simulink model "VCU_tb"  (R2023b)
settings: Solver=ode8  StartTime=0.0  StopTime=inf  FixedStep=0.0001  RelTol=1e-3
undefined symbols (not defined in the file or in its folder): canChannel
libraries: fl_lib x3, nesl_utility x3, ee_lib x2, canmsglib x1, canlib x1
settings Model: Creator=rebek  LastModifiedBy=heyka

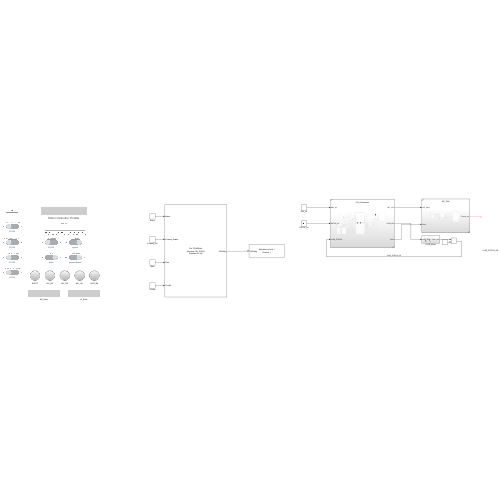
[thumbnail: Simulink's stored preview of the top-level diagram]
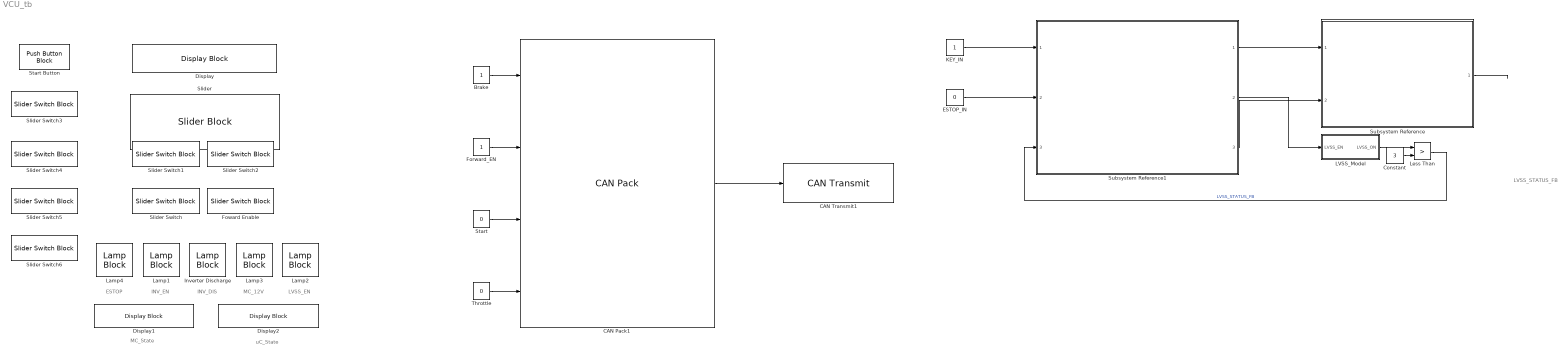
== system VCU_tb ==
  note: MC_State
  note: LVSS_EN
  note: INV_EN
  note: INV_DIS
  note: LVSS_STATUS_FB
  note: MC_12V
  note: uC_State
  note: ESTOP
  Brake : Constant
  CAN Pack1 : canmsglib/CAN Pack  CANdbFile=C:\Users\heyka\MATLAB\Projects\VCU_C\PRJDB.dbc  MsgList=N8_TPDO0  MsgName=N8_TPDO0  MsgIDType=Standard (11-bit identifier)  MsgIdentifier=392  MsgLength=5  Remote=off  ApplyMinMax=off  BusOutput=off  SignalInfo={'Brake','1','16','LE','signed','Standard','0','1','0','0','494967295';'Forward_Enable','0','1','LE','unsigned','Standard','0','1','0','0','494967295';'Start','17','1','LE','unsigned','Standard','0','1','0','-Inf','Inf';'Throttle','18','16','LE','signed','Standard','0','1','0','-32768','32767'}
      settings: LibrarySourceBlock=canlib/CAN Pack  DataFormat=CANdb specified signals
  CAN Transmit1 : canlib/CAN Transmit  BlockHandle=4.0001  Device=MathWorks Virtual 1 (Channel 1)  DeviceMenu=MathWorks Virtual 1 (Channel 1)  ObjConstructor=canChannel('MathWorks', 'Virtual 1', 1)  EnableEventTransmit=off  EnablePeriodicTransmit=off  MessagePeriod=1.000
  Constant : Constant  Value=3
  Display : DisplayBlock  LabelPosition=Hide  Transparency=1
      settings: AttributesFormatString=Motor Controller Throttle
  Display1 : DisplayBlock  LabelPosition=Hide  Transparency=1
  Display2 : DisplayBlock  LabelPosition=Hide  Transparency=1
  ESTOP_IN : Constant  Value=0
  Forward_EN : Constant
  Foward Enable : SliderSwitchBlock
      settings: Values={{'Off', 'On'}, [0 1]}
      settings: AttributesFormatString=Forward Enable
  Inverter Discharge : LampBlock  LabelPosition=Hide
  KEY_IN : Constant
  LVSS_Model : Subsystem
  Lamp{1..4} (4 alike) : LampBlock  LabelPosition=Hide
  Less Than : RelationalOperator  Operator=>  OutDataTypeStr=boolean  RndMeth=Simplest  InputSameDT=off
  Slider : SliderBlock  ScaleMax=4000
  Slider Switch{,1..6} (7 alike) : SliderSwitchBlock
      settings: Values={{'Off', 'On'}, [0 1]}
      Slider Switch settings: AttributesFormatString=Brake
      Slider Switch1 settings: AttributesFormatString=ESTOP
      Slider Switch2 settings: AttributesFormatString=Ignition
      Slider Switch3 settings: AttributesFormatString=ESTOP
      Slider Switch4 settings: AttributesFormatString=ESTOP
      Slider Switch5 settings: AttributesFormatString=ESTOP
      Slider Switch6 settings: AttributesFormatString=ESTOP
  Start : Constant  Value=0
  Start Button : PushButtonBlock  ButtonText=Start  OffValue=0.000000
  Subsystem Reference : Subsystem  ReferencedSubsystem=MC_CAN
  Subsystem Reference1 : Subsystem  ReferencedSubsystem=VCU_Subsystem
  Throttle : Constant  Value=0
  wires:
  ESTOP_IN/1 -> Subsystem Reference1/2
  KEY_IN/1 -> Subsystem Reference1/1
  CAN Pack1/1 -> CAN Transmit1/1
  Forward_EN/1 -> CAN Pack1/2
  Throttle/1 -> CAN Pack1/4
  Start/1 -> CAN Pack1/3
  Brake/1 -> CAN Pack1/1
  Subsystem Reference1/2 -> LVSS_Model/1(LVSS_EN)
  LVSS_Model/1(LVSS_ON) -> Less Than/1
  Constant/1 -> Less Than/2
  Less Than/1 -> Subsystem Reference1/3  "LVSS_STATUS_FB"
  Subsystem Reference1/1 -> Subsystem Reference/1
  Subsystem Reference/1 -> ?
  Subsystem Reference1/3 -> Subsystem Reference/2

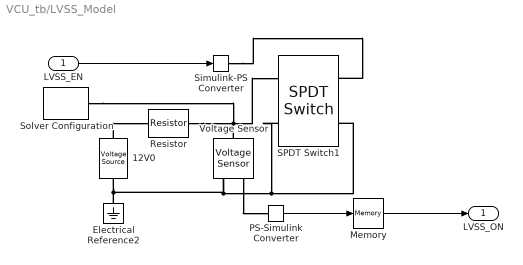
== system VCU_tb/LVSS_Model ==
  LVSS_EN : Inport
  12V0 : ee_lib/Sources/Voltage Source  dc_voltage=3.3 V  ac_voltage=0 V  ac_shift=0 rad  ac_frequency=60 Hz  noise_mode=ee.enum.sources.noise.Disabled  PSD=0 V^2/Hz  sample_time=1e-3 s  repeatability=ee.enum.sources.repeatability.NotRepeatable  user_seed=0  auto_seed=3499211588  i_specify=off  i_priority=None  i=0 A  i_nominal_specify=off  i_nominal_unit=A  i_nominal_value=1  v_specify=off  v_priority=None  v=0 V  v_nominal_specify=off  v_nominal_unit=V  v_nominal_value=1
  Electrical Reference2 : fl_lib/Electrical/Electrical Elements/Electrical Reference
  Memory : Memory
  PS-Simulink Converter : nesl_utility/PS-Simulink Converter  PhysicalDomain=network_engine_domain  SubClassName=ps_output  LeftPortType=input  RightPortType=output  PseudoPeriodic=off  Frequencies=[]  VectorFormat=inherit  Unit=inherit  AffineConversion=off
  Resistor : fl_lib/Electrical/Electrical Elements/Resistor  R=10000 Ohm  i_specify=off  i_priority=None  i=0 A  i_nominal_specify=off  i_nominal_unit=A  i_nominal_value=1  v_specify=off  v_priority=None  v=0 V  v_nominal_specify=off  v_nominal_unit=V  v_nominal_value=1
  SPDT Switch1 : ee_lib/Switches & Breakers/SPDT Switch  R_closed=0.01 Ohm  G_open=1e-10 S  Threshold=0.5 V  Width=0 V  model_dynamics=0  t_on=1e-3 s  t_off=1e-3 s  initial_vT=0 V
  Simulink-PS Converter : nesl_utility/Simulink-PS Converter  PhysicalDomain=network_engine_domain  SubClassName=ps_input  LeftPortType=input  RightPortType=output  PseudoPeriodic=off  Frequencies=[]  NoiseDistribution=none  NoiseParameters=[]  Unit=1  AffineConversion=off  FilteringAndDerivatives=provide  SimscapeFilterOrder=1  InputFilterTimeConstant=0.001  UdotUserProvided=0
  Solver Configuration : nesl_utility/Solver Configuration  PhysicalDomain=network_engine_domain  SubClassName=solver  LeftPortType=input  RightPortType=generic  Tones=[]  Harmonics=[]  SimulateNoise=off  Profile=off  UseLocalSampling=off  EnableSwitchedLinearOptims=on  FrequencyDomain=off  UseCCode=off  RelTol=0.001  AbsTol=0.001  MinStep=1e-09  ToWorkspace=off  RevertToSquareIcSolve=off  NumHomotopyIterations=100  PhasorMode=off  PhasorModeNumHarmonics=1  ConsistencySolver=NEWTON_XTOL_AFTER_FTOL  IndexReductionMethod=DerivativeReplacement  DoDC=off  ResidualTolerance=1e-09  ConsistencyTolSource=GLOBAL  ConsistencyAbsTol=0.001  ConsistencyRelTol=0.001  ConsistencyTolFactor=0.001  UseLocalSolver=off  LocalSolverChoice=NE_BACKWARD_EULER_ADVANCER  ResolveIndetEquations=on  FunctionEvalNumThread=1  LocalSolverSampleTime=0.001  DoFixedCost=off  MaxNonlinIter=3  MaxModeIter=2  ComputeImpulses=off  ImpulseIterations=2  LinearAlgebra=auto  LinearAlgebraNumThread=0  EquationFormulation=NE_TIME_EF  DelaysMemoryBudget=1024  AutomaticFiltering=on  FilteringTimeConstant=0.001  PartitionStorageMethod=AS_NEEDED  PartitionMemoryBudget=1024  PartitionMethod=ROBUST  MultibodyUseLocalSolver=off  MultibodyLocalSolverChoice=ODE1  MultibodyLocalSolverSampleTime=0.001
  Voltage Sensor : fl_lib/Electrical/Electrical Sensors/Voltage Sensor
  LVSS_ON : Outport
  wires:
  LVSS_EN/1 -> Simulink-PS Converter/1
  PS-Simulink Converter/1 -> Memory/1
  Memory/1 -> LVSS_ON/1
  connections:
  Electrical Reference2/LConn1 -- SPDT Switch1/RConn2 -- SPDT Switch1/LConn2 -- Voltage Sensor/RConn2 -- 12V0/RConn1
  Solver Configuration/RConn1 -- Voltage Sensor/LConn1 -- SPDT Switch1/RConn1 -- Resistor/RConn1
  Simulink-PS Converter/RConn1 -- SPDT Switch1/LConn1
  Voltage Sensor/RConn1 -- PS-Simulink Converter/LConn1
  12V0/LConn1 -- Resistor/LConn1
